simulink model "sim_tcyb_2024_pos_ctrl"  (R2020a)
settings: Solver=ode4  StartTime=0.0  StopTime=30.0  FixedStep=0.01  RelTol=1e-3
values from neighbouring files (symbols this model uses):
  alfa_theta = 20    [init_tcyb_2024_pos_ctrl.m]
  alfa_theta_obs = 100    [init_tcyb_2024_pos_ctrl.m]
  c1_diff_sigma_bar_v = diag([25; 30; 20])    [init_tcyb_2024_pos_ctrl.m]
  c1v = diag([5.8; 6.5; 6.5])    [init_tcyb_2024_pos_ctrl.m]
  c2_diff_sigma_bar_v = diag([50; 50; 10])    [init_tcyb_2024_pos_ctrl.m]
  c2v = diag([5.8; 6.5; 6.5])    [init_tcyb_2024_pos_ctrl.m]
  c3_diff_sigma_bar_v = diag([15; 15; 10])    [init_tcyb_2024_pos_ctrl.m]
  c3v = diag([4.8; 6.4; 6.0])    [init_tcyb_2024_pos_ctrl.m]
  c_psi_p = [0.05; 0.05; 0.05]    [init_tcyb_2024_pos_ctrl.m]
  delta_p_i_0 = zeros(3, NF)    [init_tcyb_2024_pos_ctrl.m]
  delta_v_i_0 = zeros(3, NF)    [init_tcyb_2024_pos_ctrl.m]
  dp_aa_t = 0.2 * ones(3, 5) + ( 1.0 - 0.2 ) * rand(3, 5)    [init_tcyb_2024_pos_ctrl.m]
  dp_ff_t = [ 0.4 * ones(1, 5) + ( 1.0 - 0.4 ) * rand(1, 5);                      0.4 * ones(1, 5) + ( 1.0 - 0.4 ) * rand(1, 5);                      0.2 * ones(1, 5) + ( 0.6 - 0.2 ) * rand(1, 5) ]    [init_tcyb_2024_pos_ctrl.m]
  dp_phi_t = ( - pi / 2 ) * ones(3, 5) + ( pi / 2 - ( - pi / 2 ) ) * rand(3, 5)    [init_tcyb_2024_pos_ctrl.m]
  etai_0 = zeros(3,5)    [init_tcyb_2024_pos_ctrl.m]
  kai_1_t = 0.02    [init_tcyb_2024_pos_ctrl.m]
  kai_3_t = 0.1    [init_tcyb_2024_pos_ctrl.m]
  ksii_0 = zeros(3,5)    [init_tcyb_2024_pos_ctrl.m]
  l1v = diag([20; 20; 20])    [init_tcyb_2024_pos_ctrl.m]
  l2v = diag([30; 30; 30])    [init_tcyb_2024_pos_ctrl.m]
  Lamd_diff_sigma_bar_v = 0.5    [init_tcyb_2024_pos_ctrl.m]
  mass_i = zeros(1,NF)    [init_tcyb_2024_pos_ctrl.m]
  Mii = diag([1;0;0;0;1])    [init_tcyb_2024_pos_ctrl.m]
  pos0 = zeros(3, 1)    [init_tcyb_2024_pos_ctrl.m]
  PZ0 = P0(3)    [init_tcyb_2024_pos_ctrl.m]
  PZ1 = 10    [init_tcyb_2024_pos_ctrl.m]
  Qci_init = repmat([1;0;0;0],1,NF)    [init_tcyb_2024_pos_ctrl.m]
  R0 = 4    [init_tcyb_2024_pos_ctrl.m]
  R1 = 8    [init_tcyb_2024_pos_ctrl.m]
  rho_p = [0.1; 0.1; 0.1]    [init_tcyb_2024_pos_ctrl.m]
  Rx2 = 10    [init_tcyb_2024_pos_ctrl.m]
  Ry2 = 6    [init_tcyb_2024_pos_ctrl.m]
  Rz2 = 4    [init_tcyb_2024_pos_ctrl.m]
  T0 = 0    [init_tcyb_2024_pos_ctrl.m]
  T1 = tseq1    (= 10)    [init_tcyb_2024_pos_ctrl.m]
  T12 = tseq1 + tseq12    (= 20)    [init_tcyb_2024_pos_ctrl.m]
  T2 = tseq1 + tseq12 + tseq2    (= 30)    [init_tcyb_2024_pos_ctrl.m]
  tau_p = 5    [init_tcyb_2024_pos_ctrl.m]
  theta0 = ( 2 / 5 ) * pi    (= 1.25663706144)    [init_tcyb_2024_pos_ctrl.m]
  vel0 = zeros(3, 1)    [init_tcyb_2024_pos_ctrl.m]
  Wij = [0,0,1,0,0;              0,0,1,1,0;              1,0,0,0,1;              0,1,1,0,0;              0,0,1,0,0]    [init_tcyb_2024_pos_ctrl.m]
  X1 = 8    [init_tcyb_2024_pos_ctrl.m]
  X2 = 2    [init_tcyb_2024_pos_ctrl.m]
  X3 = 3    [init_tcyb_2024_pos_ctrl.m]
  Y1 = 10    [init_tcyb_2024_pos_ctrl.m]
  Y2 = 2    [init_tcyb_2024_pos_ctrl.m]
  Y3 = 4    [init_tcyb_2024_pos_ctrl.m]
  Z1 = 4    [init_tcyb_2024_pos_ctrl.m]
  Z2 = -6    [init_tcyb_2024_pos_ctrl.m]
  Z3 = 2    [init_tcyb_2024_pos_ctrl.m]
  zeta_diff_sigma_bar_v = 0.08    [init_tcyb_2024_pos_ctrl.m]
undefined symbols (not defined in the file or in its folder): cal_frac_squ, p_alfav1, p_alfav2, p_gamma1_pos, p_gamma1_vel, p_gamma2_pos, p_gamma2_vel, q_alfav1, q_alfav2, q_gamma1_pos, q_gamma1_vel, q_gamma2_pos, q_gamma2_vel
(part 2 of 4)

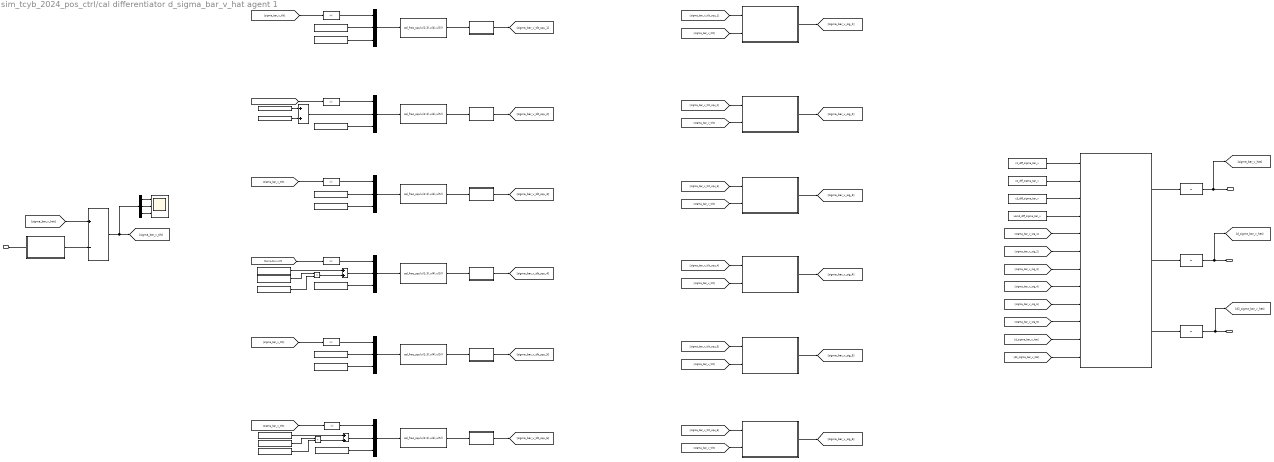
== system sim_tcyb_2024_pos_ctrl/cal differentiator d_sigma_bar_v_hat agent 1 ==
  x : Inport
  Abs{,1..5} (6 alike) : Abs
  Add : Sum
  Add1 : Sum
  Add2 : Sum
  Add3 : Sum  Inputs=+-
  Constant : Constant  Value=0
  Constant{97,100,105,107,109} (5 alike) : Constant
  Constant{98..99,101,108,110..111} (6 alike) : Constant  Value=3
  Constant102 : Constant  Value=2
  Constant103 : Constant  Value=c1_diff_sigma_bar_v
  Constant104 : Constant  Value=c2_diff_sigma_bar_v
  Constant106 : Constant  Value=c3_diff_sigma_bar_v
  Constant112 : Constant  Value=2
  Constant113 : Constant  Value=Lamd_diff_sigma_bar_v
  Constant161 : Constant  Value=zeta_diff_sigma_bar_v
  Constant162 : Constant  Value=zeta_diff_sigma_bar_v
  Constant163 : Constant  Value=zeta_diff_sigma_bar_v
  Demux2 : Demux  Outputs=3
  Integrator2 : Integrator  InitialCondition=zeros(3,1)
  Integrator3 : Integrator  InitialCondition=zeros(3,1)
  Integrator4 : Integrator  InitialCondition=zeros(3,1)
  Interpreted MATLAB Function{,20..24} (6 alike) : MATLABFcn  MATLABFcn=cal_frac_squ(u(1:3),u(4),u(5))
  Mux{19..24} (6 alike) : Mux  Inputs=3
  Product : Product
  Product1 : Product
  cal differentiator : MATLAB Function  TreatAsAtomicUnit=on
  cal sig : MATLAB Function  TreatAsAtomicUnit=on
  cal sig1 : MATLAB Function  TreatAsAtomicUnit=on
  cal sig2 : MATLAB Function  TreatAsAtomicUnit=on
  cal sig3 : MATLAB Function  TreatAsAtomicUnit=on
  cal sig4 : MATLAB Function  TreatAsAtomicUnit=on
  cal sig5 : MATLAB Function  TreatAsAtomicUnit=on
  choose sigma_bar_v : MATLAB Function  TreatAsAtomicUnit=on
  sigma_bar_v_tilt : Scope  NumInputPorts=3
  trans to column20 : MATLAB Function  TreatAsAtomicUnit=on
  trans to column21 : MATLAB Function  TreatAsAtomicUnit=on
  trans to column22 : MATLAB Function  TreatAsAtomicUnit=on
  trans to column23 : MATLAB Function  TreatAsAtomicUnit=on
  trans to column24 : MATLAB Function  TreatAsAtomicUnit=on
  trans to column25 : MATLAB Function  TreatAsAtomicUnit=on
  Out1 : Outport
  Out2 : Outport  Port=2
  Out3 : Outport  Port=3
  wires:
  Abs/1 -> Mux22/1
  [sigma_bar_v_tilt] -> cal sig/2(y)
  cal sig1/1(z) -> [sigma_bar_v_sig_2]
  [d2_sigma_bar_v_hat] -> cal differentiator/12(d2_sigma_bar_v_hat)
  trans to column23/1(y) -> [sigma_bar_v_tilt_squ_3]
  Add/1 -> Mux21/2
  Demux2/1 -> sigma_bar_v_tilt/1
  [sigma_bar_v_tilt] -> cal sig4/2(y)
  Product1/1 -> Add2/2
  Add2/1 -> Mux19/2
  [d_sigma_bar_v_hat] -> cal differentiator/11("d_sigma_bar_v_hat ")
  [sigma_bar_v_sig_3] -> cal differentiator/7(sigma_bar_v_sig_3)
  trans to column24/1(y) -> [sigma_bar_v_tilt_squ_4]
  Constant107/1 -> Mux21/3
  [sigma_bar_v_sig_5] -> cal differentiator/9(sigma_bar_v_sig_5)
  Constant97/1 -> Mux22/3
  cal sig/1(z) -> [sigma_bar_v_sig_1]
  trans to column22/1(y) -> [sigma_bar_v_tilt_squ_1]
  [sigma_bar_v_tilt_squ_3] -> cal sig2/1(x)
  [sigma_bar_v_tilt] -> Abs3/1
  Interpreted MATLAB Function24/1 -> trans to column25/1(x)
  [sigma_bar_v_sig_1] -> cal differentiator/5(sigma_bar_v_sig_1)
  cal differentiator/1(d_sigma_bar_v_hat) -> Integrator2/1
  Constant110/1 -> Mux24/3
  cal sig5/1(z) -> [sigma_bar_v_sig_5]
  [sigma_bar_v_tilt] -> Abs4/1
  Demux2/3 -> sigma_bar_v_tilt/3
  cal sig2/1(z) -> [sigma_bar_v_sig_3]
  Constant112/1 -> Product/1
  Constant/1 -> Mux22/2
  cal differentiator/3(d_d2sigma_bar_v_hat) -> Integrator4/1
  Abs3/1 -> Mux24/1
  trans to column21/1(y) -> [sigma_bar_v_tilt_squ_2]
  Constant99/1 -> Add2/1
  Constant103/1 -> cal differentiator/1(c1)
  Mux19/1 -> Interpreted MATLAB Function24/1
  [sigma_bar_v_tilt_squ_6] -> cal sig3/1(x)
  Constant106/1 -> cal differentiator/3(c3)
  [sigma_bar_v_tilt] -> Abs2/1
  [sigma_bar_v_tilt_squ_2] -> cal sig1/1(x)
  Constant162/1 -> Product/2
  Product/1 -> Add1/2
  [sigma_bar_v_sig_4] -> cal differentiator/8(sigma_bar_v_sig_4)
  [sigma_bar_v_hat] -> Add3/1
  Constant102/1 -> Mux20/2
  Add3/1 -> Demux2/1, [sigma_bar_v_tilt]
  cal differentiator/2(d_dsigma_bar_v_hat) -> Integrator3/1
  [sigma_bar_v_tilt] -> Abs5/1
  [sigma_bar_v_tilt] -> cal sig2/2(y)
  [sigma_bar_v_sig_6] -> cal differentiator/10(sigma_bar_v_sig_6)
  trans to column20/1(y) -> [sigma_bar_v_tilt_squ_5]
  Constant104/1 -> cal differentiator/2(c2)
  Constant101/1 -> Mux20/3
  Mux22/1 -> Interpreted MATLAB Function/1
  Constant163/1 -> Product1/2
  Abs2/1 -> Mux23/1
  Interpreted MATLAB Function21/1 -> trans to column21/1(x)
  Interpreted MATLAB Function23/1 -> trans to column24/1(x)
  Mux23/1 -> Interpreted MATLAB Function22/1
  cal sig3/1(z) -> [sigma_bar_v_sig_6]
  Abs4/1 -> Mux19/1
  trans to column25/1(y) -> [sigma_bar_v_tilt_squ_6]
  Constant113/1 -> cal differentiator/4(chi_t)
  choose sigma_bar_v/1(y) -> Add3/2
  Interpreted MATLAB Function/1 -> trans to column22/1(x)
  Interpreted MATLAB Function20/1 -> trans to column20/1(x)
  Constant108/1 -> Mux23/3
  [sigma_bar_v_sig_2] -> cal differentiator/6(sigma_bar_v_sig_2)
  [sigma_bar_v_tilt] -> cal sig1/2(y)
  [sigma_bar_v_tilt_squ_1] -> cal sig/1(x)
  Constant100/1 -> Product1/1
  Abs1/1 -> Mux21/1
  Demux2/2 -> sigma_bar_v_tilt/2
  Integrator4/1 -> [d2_sigma_bar_v_hat], Out3/1
  [sigma_bar_v_tilt_squ_4] -> cal sig4/1(x)
  Abs5/1 -> Mux20/1
  Constant98/1 -> Mux19/3
  Constant111/1 -> Add1/1
  [sigma_bar_v_tilt] -> cal sig5/2(y)
  Constant109/1 -> Mux23/2
  [sigma_bar_v_tilt] -> Abs/1
  Mux24/1 -> Interpreted MATLAB Function23/1
  [sigma_bar_v_tilt] -> Abs1/1
  [sigma_bar_v_tilt_squ_5] -> cal sig5/1(x)
  Add1/1 -> Mux24/2
  cal sig4/1(z) -> [sigma_bar_v_sig_4]
  Constant161/1 -> Add/2
  [sigma_bar_v_tilt] -> cal sig3/2(y)
  Mux21/1 -> Interpreted MATLAB Function21/1
  Interpreted MATLAB Function22/1 -> trans to column23/1(x)
  Mux20/1 -> Interpreted MATLAB Function20/1
  x/1 -> choose sigma_bar_v/1(x)
  Constant105/1 -> Add/1
  Integrator2/1 -> [sigma_bar_v_hat], Out1/1
  Integrator3/1 -> [d_sigma_bar_v_hat], Out2/1

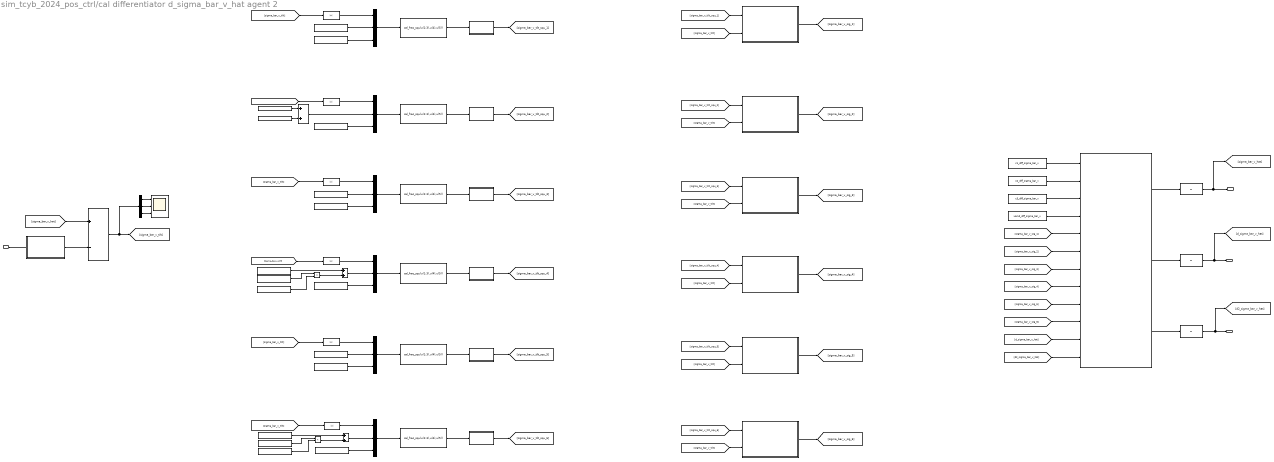
== system sim_tcyb_2024_pos_ctrl/cal differentiator d_sigma_bar_v_hat agent 2 ==
  x : Inport
  Abs{,1..5} (6 alike) : Abs
  Add : Sum
  Add1 : Sum
  Add2 : Sum
  Add3 : Sum  Inputs=+-
  Constant : Constant  Value=0
  Constant{97,100,105,107,109} (5 alike) : Constant
  Constant{98..99,101,108,110..111} (6 alike) : Constant  Value=3
  Constant102 : Constant  Value=2
  Constant103 : Constant  Value=c1_diff_sigma_bar_v
  Constant104 : Constant  Value=c2_diff_sigma_bar_v
  Constant106 : Constant  Value=c3_diff_sigma_bar_v
  Constant112 : Constant  Value=2
  Constant113 : Constant  Value=Lamd_diff_sigma_bar_v
  Constant161 : Constant  Value=zeta_diff_sigma_bar_v
  Constant162 : Constant  Value=zeta_diff_sigma_bar_v
  Constant163 : Constant  Value=zeta_diff_sigma_bar_v
  Demux2 : Demux  Outputs=3
  Integrator2 : Integrator  InitialCondition=zeros(3,1)
  Integrator3 : Integrator  InitialCondition=zeros(3,1)
  Integrator4 : Integrator  InitialCondition=zeros(3,1)
  Interpreted MATLAB Function{,20..24} (6 alike) : MATLABFcn  MATLABFcn=cal_frac_squ(u(1:3),u(4),u(5))
  Mux{19..24} (6 alike) : Mux  Inputs=3
  Product : Product
  Product1 : Product
  cal differentiator : MATLAB Function  TreatAsAtomicUnit=on
  cal sig : MATLAB Function  TreatAsAtomicUnit=on
  cal sig1 : MATLAB Function  TreatAsAtomicUnit=on
  cal sig2 : MATLAB Function  TreatAsAtomicUnit=on
  cal sig3 : MATLAB Function  TreatAsAtomicUnit=on
  cal sig4 : MATLAB Function  TreatAsAtomicUnit=on
  cal sig5 : MATLAB Function  TreatAsAtomicUnit=on
  choose sigma_bar_v : MATLAB Function  TreatAsAtomicUnit=on
  sigma_bar_v_tilt : Scope  NumInputPorts=3
  trans to column20 : MATLAB Function  TreatAsAtomicUnit=on
  trans to column21 : MATLAB Function  TreatAsAtomicUnit=on
  trans to column22 : MATLAB Function  TreatAsAtomicUnit=on
  trans to column23 : MATLAB Function  TreatAsAtomicUnit=on
  trans to column24 : MATLAB Function  TreatAsAtomicUnit=on
  trans to column25 : MATLAB Function  TreatAsAtomicUnit=on
  Out1 : Outport
  Out2 : Outport  Port=2
  Out3 : Outport  Port=3
  wires:
  Abs/1 -> Mux22/1
  [sigma_bar_v_tilt] -> cal sig/2(y)
  cal sig1/1(z) -> [sigma_bar_v_sig_2]
  [d2_sigma_bar_v_hat] -> cal differentiator/12(d2_sigma_bar_v_hat)
  trans to column23/1(y) -> [sigma_bar_v_tilt_squ_3]
  Add/1 -> Mux21/2
  Demux2/1 -> sigma_bar_v_tilt/1
  [sigma_bar_v_tilt] -> cal sig4/2(y)
  Product1/1 -> Add2/2
  Add2/1 -> Mux19/2
  [d_sigma_bar_v_hat] -> cal differentiator/11("d_sigma_bar_v_hat ")
  [sigma_bar_v_sig_3] -> cal differentiator/7(sigma_bar_v_sig_3)
  trans to column24/1(y) -> [sigma_bar_v_tilt_squ_4]
  Constant107/1 -> Mux21/3
  [sigma_bar_v_sig_5] -> cal differentiator/9(sigma_bar_v_sig_5)
  Constant97/1 -> Mux22/3
  cal sig/1(z) -> [sigma_bar_v_sig_1]
  trans to column22/1(y) -> [sigma_bar_v_tilt_squ_1]
  [sigma_bar_v_tilt_squ_3] -> cal sig2/1(x)
  [sigma_bar_v_tilt] -> Abs3/1
  Interpreted MATLAB Function24/1 -> trans to column25/1(x)
  [sigma_bar_v_sig_1] -> cal differentiator/5(sigma_bar_v_sig_1)
  cal differentiator/1(d_sigma_bar_v_hat) -> Integrator2/1
  Constant110/1 -> Mux24/3
  cal sig5/1(z) -> [sigma_bar_v_sig_5]
  [sigma_bar_v_tilt] -> Abs4/1
  Demux2/3 -> sigma_bar_v_tilt/3
  cal sig2/1(z) -> [sigma_bar_v_sig_3]
  Constant112/1 -> Product/1
  Constant/1 -> Mux22/2
  cal differentiator/3(d_d2sigma_bar_v_hat) -> Integrator4/1
  Abs3/1 -> Mux24/1
  trans to column21/1(y) -> [sigma_bar_v_tilt_squ_2]
  Constant99/1 -> Add2/1
  Constant103/1 -> cal differentiator/1(c1)
  Mux19/1 -> Interpreted MATLAB Function24/1
  [sigma_bar_v_tilt_squ_6] -> cal sig3/1(x)
  Constant106/1 -> cal differentiator/3(c3)
  [sigma_bar_v_tilt] -> Abs2/1
  [sigma_bar_v_tilt_squ_2] -> cal sig1/1(x)
  Constant162/1 -> Product/2
  Product/1 -> Add1/2
  [sigma_bar_v_sig_4] -> cal differentiator/8(sigma_bar_v_sig_4)
  [sigma_bar_v_hat] -> Add3/1
  Constant102/1 -> Mux20/2
  Add3/1 -> Demux2/1, [sigma_bar_v_tilt]
  cal differentiator/2(d_dsigma_bar_v_hat) -> Integrator3/1
  [sigma_bar_v_tilt] -> Abs5/1
  [sigma_bar_v_tilt] -> cal sig2/2(y)
  [sigma_bar_v_sig_6] -> cal differentiator/10(sigma_bar_v_sig_6)
  trans to column20/1(y) -> [sigma_bar_v_tilt_squ_5]
  Constant104/1 -> cal differentiator/2(c2)
  Constant101/1 -> Mux20/3
  Mux22/1 -> Interpreted MATLAB Function/1
  Constant163/1 -> Product1/2
  Abs2/1 -> Mux23/1
  Interpreted MATLAB Function21/1 -> trans to column21/1(x)
  Interpreted MATLAB Function23/1 -> trans to column24/1(x)
  Mux23/1 -> Interpreted MATLAB Function22/1
  cal sig3/1(z) -> [sigma_bar_v_sig_6]
  Abs4/1 -> Mux19/1
  trans to column25/1(y) -> [sigma_bar_v_tilt_squ_6]
  Constant113/1 -> cal differentiator/4(chi_t)
  choose sigma_bar_v/1(y) -> Add3/2
  Interpreted MATLAB Function/1 -> trans to column22/1(x)
  Interpreted MATLAB Function20/1 -> trans to column20/1(x)
  Constant108/1 -> Mux23/3
  [sigma_bar_v_sig_2] -> cal differentiator/6(sigma_bar_v_sig_2)
  [sigma_bar_v_tilt] -> cal sig1/2(y)
  [sigma_bar_v_tilt_squ_1] -> cal sig/1(x)
  Constant100/1 -> Product1/1
  Abs1/1 -> Mux21/1
  Demux2/2 -> sigma_bar_v_tilt/2
  Integrator4/1 -> [d2_sigma_bar_v_hat], Out3/1
  [sigma_bar_v_tilt_squ_4] -> cal sig4/1(x)
  Abs5/1 -> Mux20/1
  Constant98/1 -> Mux19/3
  Constant111/1 -> Add1/1
  [sigma_bar_v_tilt] -> cal sig5/2(y)
  Constant109/1 -> Mux23/2
  [sigma_bar_v_tilt] -> Abs/1
  Mux24/1 -> Interpreted MATLAB Function23/1
  [sigma_bar_v_tilt] -> Abs1/1
  [sigma_bar_v_tilt_squ_5] -> cal sig5/1(x)
  Add1/1 -> Mux24/2
  cal sig4/1(z) -> [sigma_bar_v_sig_4]
  Constant161/1 -> Add/2
  [sigma_bar_v_tilt] -> cal sig3/2(y)
  Mux21/1 -> Interpreted MATLAB Function21/1
  Interpreted MATLAB Function22/1 -> trans to column23/1(x)
  Mux20/1 -> Interpreted MATLAB Function20/1
  x/1 -> choose sigma_bar_v/1(x)
  Constant105/1 -> Add/1
  Integrator2/1 -> [sigma_bar_v_hat], Out1/1
  Integrator3/1 -> [d_sigma_bar_v_hat], Out2/1

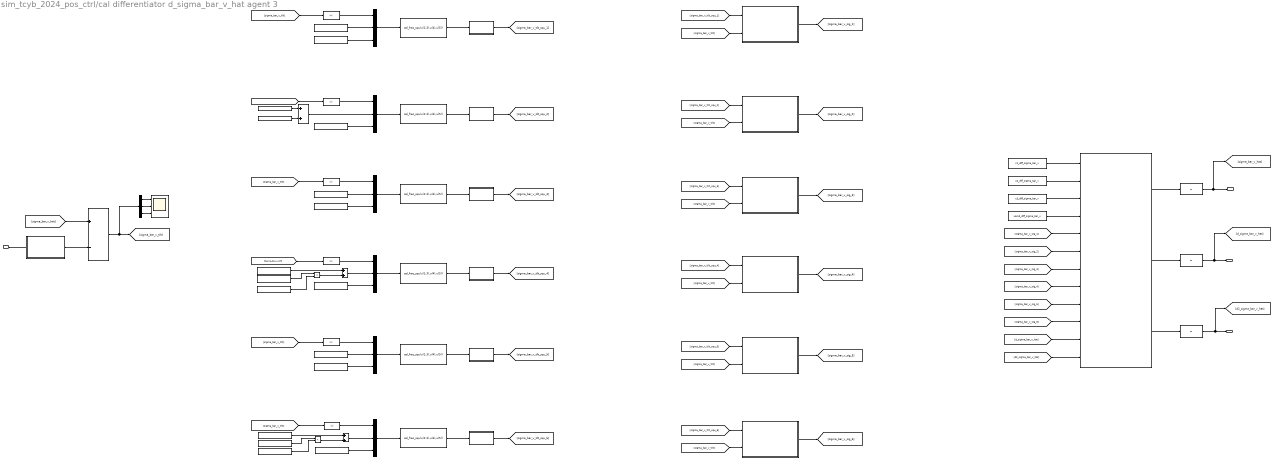
== system sim_tcyb_2024_pos_ctrl/cal differentiator d_sigma_bar_v_hat agent 3 ==
  x : Inport
  Abs{,1..5} (6 alike) : Abs
  Add : Sum
  Add1 : Sum
  Add2 : Sum
  Add3 : Sum  Inputs=+-
  Constant : Constant  Value=0
  Constant{97,100,105,107,109} (5 alike) : Constant
  Constant{98..99,101,108,110..111} (6 alike) : Constant  Value=3
  Constant102 : Constant  Value=2
  Constant103 : Constant  Value=c1_diff_sigma_bar_v
  Constant104 : Constant  Value=c2_diff_sigma_bar_v
  Constant106 : Constant  Value=c3_diff_sigma_bar_v
  Constant112 : Constant  Value=2
  Constant113 : Constant  Value=Lamd_diff_sigma_bar_v
  Constant161 : Constant  Value=zeta_diff_sigma_bar_v
  Constant162 : Constant  Value=zeta_diff_sigma_bar_v
  Constant163 : Constant  Value=zeta_diff_sigma_bar_v
  Demux2 : Demux  Outputs=3
  Integrator2 : Integrator  InitialCondition=zeros(3,1)
  Integrator3 : Integrator  InitialCondition=zeros(3,1)
  Integrator4 : Integrator  InitialCondition=zeros(3,1)
  Interpreted MATLAB Function{,20..24} (6 alike) : MATLABFcn  MATLABFcn=cal_frac_squ(u(1:3),u(4),u(5))
  Mux{19..24} (6 alike) : Mux  Inputs=3
  Product : Product
  Product1 : Product
  cal differentiator : MATLAB Function  TreatAsAtomicUnit=on
  cal sig : MATLAB Function  TreatAsAtomicUnit=on
  cal sig1 : MATLAB Function  TreatAsAtomicUnit=on
  cal sig2 : MATLAB Function  TreatAsAtomicUnit=on
  cal sig3 : MATLAB Function  TreatAsAtomicUnit=on
  cal sig4 : MATLAB Function  TreatAsAtomicUnit=on
  cal sig5 : MATLAB Function  TreatAsAtomicUnit=on
  choose sigma_bar_v : MATLAB Function  TreatAsAtomicUnit=on
  sigma_bar_v_tilt : Scope  NumInputPorts=3
  trans to column20 : MATLAB Function  TreatAsAtomicUnit=on
  trans to column21 : MATLAB Function  TreatAsAtomicUnit=on
  trans to column22 : MATLAB Function  TreatAsAtomicUnit=on
  trans to column23 : MATLAB Function  TreatAsAtomicUnit=on
  trans to column24 : MATLAB Function  TreatAsAtomicUnit=on
  trans to column25 : MATLAB Function  TreatAsAtomicUnit=on
  Out1 : Outport
  Out2 : Outport  Port=2
  Out3 : Outport  Port=3
  wires:
  Abs/1 -> Mux22/1
  [sigma_bar_v_tilt] -> cal sig/2(y)
  cal sig1/1(z) -> [sigma_bar_v_sig_2]
  [d2_sigma_bar_v_hat] -> cal differentiator/12(d2_sigma_bar_v_hat)
  trans to column23/1(y) -> [sigma_bar_v_tilt_squ_3]
  Add/1 -> Mux21/2
  Demux2/1 -> sigma_bar_v_tilt/1
  [sigma_bar_v_tilt] -> cal sig4/2(y)
  Product1/1 -> Add2/2
  Add2/1 -> Mux19/2
  [d_sigma_bar_v_hat] -> cal differentiator/11("d_sigma_bar_v_hat ")
  [sigma_bar_v_sig_3] -> cal differentiator/7(sigma_bar_v_sig_3)
  trans to column24/1(y) -> [sigma_bar_v_tilt_squ_4]
  Constant107/1 -> Mux21/3
  [sigma_bar_v_sig_5] -> cal differentiator/9(sigma_bar_v_sig_5)
  Constant97/1 -> Mux22/3
  cal sig/1(z) -> [sigma_bar_v_sig_1]
  trans to column22/1(y) -> [sigma_bar_v_tilt_squ_1]
  [sigma_bar_v_tilt_squ_3] -> cal sig2/1(x)
  [sigma_bar_v_tilt] -> Abs3/1
  Interpreted MATLAB Function24/1 -> trans to column25/1(x)
  [sigma_bar_v_sig_1] -> cal differentiator/5(sigma_bar_v_sig_1)
  cal differentiator/1(d_sigma_bar_v_hat) -> Integrator2/1
  Constant110/1 -> Mux24/3
  cal sig5/1(z) -> [sigma_bar_v_sig_5]
  [sigma_bar_v_tilt] -> Abs4/1
  Demux2/3 -> sigma_bar_v_tilt/3
  cal sig2/1(z) -> [sigma_bar_v_sig_3]
  Constant112/1 -> Product/1
  Constant/1 -> Mux22/2
  cal differentiator/3(d_d2sigma_bar_v_hat) -> Integrator4/1
  Abs3/1 -> Mux24/1
  trans to column21/1(y) -> [sigma_bar_v_tilt_squ_2]
  Constant99/1 -> Add2/1
  Constant103/1 -> cal differentiator/1(c1)
  Mux19/1 -> Interpreted MATLAB Function24/1
  [sigma_bar_v_tilt_squ_6] -> cal sig3/1(x)
  Constant106/1 -> cal differentiator/3(c3)
  [sigma_bar_v_tilt] -> Abs2/1
  [sigma_bar_v_tilt_squ_2] -> cal sig1/1(x)
  Constant162/1 -> Product/2
  Product/1 -> Add1/2
  [sigma_bar_v_sig_4] -> cal differentiator/8(sigma_bar_v_sig_4)
  [sigma_bar_v_hat] -> Add3/1
  Constant102/1 -> Mux20/2
  Add3/1 -> Demux2/1, [sigma_bar_v_tilt]
  cal differentiator/2(d_dsigma_bar_v_hat) -> Integrator3/1
  [sigma_bar_v_tilt] -> Abs5/1
  [sigma_bar_v_tilt] -> cal sig2/2(y)
  [sigma_bar_v_sig_6] -> cal differentiator/10(sigma_bar_v_sig_6)
  trans to column20/1(y) -> [sigma_bar_v_tilt_squ_5]
  Constant104/1 -> cal differentiator/2(c2)
  Constant101/1 -> Mux20/3
  Mux22/1 -> Interpreted MATLAB Function/1
  Constant163/1 -> Product1/2
  Abs2/1 -> Mux23/1
  Interpreted MATLAB Function21/1 -> trans to column21/1(x)
  Interpreted MATLAB Function23/1 -> trans to column24/1(x)
  Mux23/1 -> Interpreted MATLAB Function22/1
  cal sig3/1(z) -> [sigma_bar_v_sig_6]
  Abs4/1 -> Mux19/1
  trans to column25/1(y) -> [sigma_bar_v_tilt_squ_6]
  Constant113/1 -> cal differentiator/4(chi_t)
  choose sigma_bar_v/1(y) -> Add3/2
  Interpreted MATLAB Function/1 -> trans to column22/1(x)
  Interpreted MATLAB Function20/1 -> trans to column20/1(x)
  Constant108/1 -> Mux23/3
  [sigma_bar_v_sig_2] -> cal differentiator/6(sigma_bar_v_sig_2)
  [sigma_bar_v_tilt] -> cal sig1/2(y)
  [sigma_bar_v_tilt_squ_1] -> cal sig/1(x)
  Constant100/1 -> Product1/1
  Abs1/1 -> Mux21/1
  Demux2/2 -> sigma_bar_v_tilt/2
  Integrator4/1 -> [d2_sigma_bar_v_hat], Out3/1
  [sigma_bar_v_tilt_squ_4] -> cal sig4/1(x)
  Abs5/1 -> Mux20/1
  Constant98/1 -> Mux19/3
  Constant111/1 -> Add1/1
  [sigma_bar_v_tilt] -> cal sig5/2(y)
  Constant109/1 -> Mux23/2
  [sigma_bar_v_tilt] -> Abs/1
  Mux24/1 -> Interpreted MATLAB Function23/1
  [sigma_bar_v_tilt] -> Abs1/1
  [sigma_bar_v_tilt_squ_5] -> cal sig5/1(x)
  Add1/1 -> Mux24/2
  cal sig4/1(z) -> [sigma_bar_v_sig_4]
  Constant161/1 -> Add/2
  [sigma_bar_v_tilt] -> cal sig3/2(y)
  Mux21/1 -> Interpreted MATLAB Function21/1
  Interpreted MATLAB Function22/1 -> trans to column23/1(x)
  Mux20/1 -> Interpreted MATLAB Function20/1
  x/1 -> choose sigma_bar_v/1(x)
  Constant105/1 -> Add/1
  Integrator2/1 -> [sigma_bar_v_hat], Out1/1
  Integrator3/1 -> [d_sigma_bar_v_hat], Out2/1

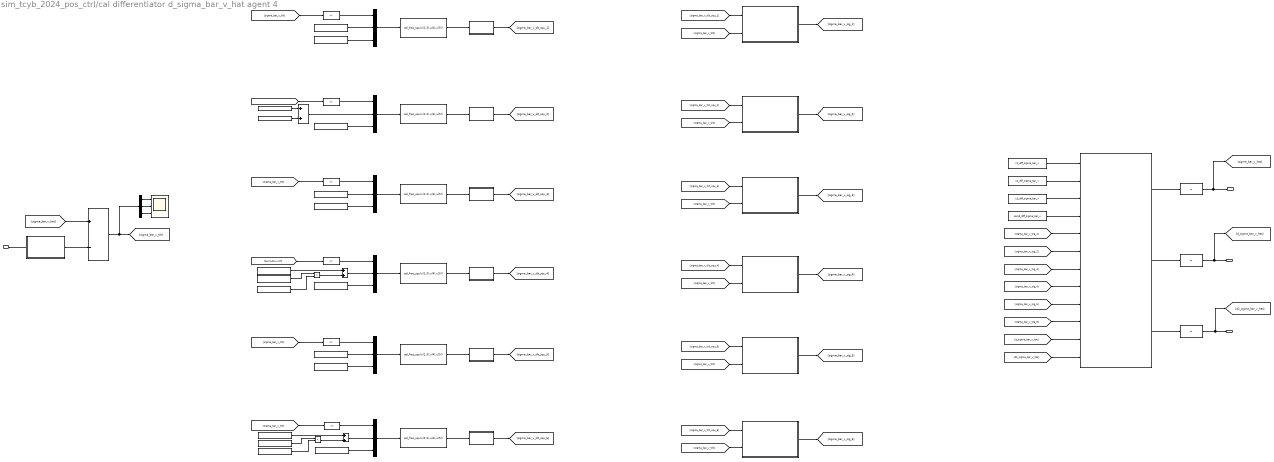
== system sim_tcyb_2024_pos_ctrl/cal differentiator d_sigma_bar_v_hat agent 4 ==
  x : Inport
  Abs{,1..5} (6 alike) : Abs
  Add : Sum
  Add1 : Sum
  Add2 : Sum
  Add3 : Sum  Inputs=+-
  Constant : Constant  Value=0
  Constant{97,100,105,107,109} (5 alike) : Constant
  Constant{98..99,101,108,110..111} (6 alike) : Constant  Value=3
  Constant102 : Constant  Value=2
  Constant103 : Constant  Value=c1_diff_sigma_bar_v
  Constant104 : Constant  Value=c2_diff_sigma_bar_v
  Constant106 : Constant  Value=c3_diff_sigma_bar_v
  Constant112 : Constant  Value=2
  Constant113 : Constant  Value=Lamd_diff_sigma_bar_v
  Constant161 : Constant  Value=zeta_diff_sigma_bar_v
  Constant162 : Constant  Value=zeta_diff_sigma_bar_v
  Constant163 : Constant  Value=zeta_diff_sigma_bar_v
  Demux2 : Demux  Outputs=3
  Integrator2 : Integrator  InitialCondition=zeros(3,1)
  Integrator3 : Integrator  InitialCondition=zeros(3,1)
  Integrator4 : Integrator  InitialCondition=zeros(3,1)
  Interpreted MATLAB Function{,20..24} (6 alike) : MATLABFcn  MATLABFcn=cal_frac_squ(u(1:3),u(4),u(5))
  Mux{19..24} (6 alike) : Mux  Inputs=3
  Product : Product
  Product1 : Product
  cal differentiator : MATLAB Function  TreatAsAtomicUnit=on
  cal sig : MATLAB Function  TreatAsAtomicUnit=on
  cal sig1 : MATLAB Function  TreatAsAtomicUnit=on
  cal sig2 : MATLAB Function  TreatAsAtomicUnit=on
  cal sig3 : MATLAB Function  TreatAsAtomicUnit=on
  cal sig4 : MATLAB Function  TreatAsAtomicUnit=on
  cal sig5 : MATLAB Function  TreatAsAtomicUnit=on
  choose sigma_bar_v : MATLAB Function  TreatAsAtomicUnit=on
  sigma_bar_v_tilt : Scope  NumInputPorts=3
  trans to column20 : MATLAB Function  TreatAsAtomicUnit=on
  trans to column21 : MATLAB Function  TreatAsAtomicUnit=on
  trans to column22 : MATLAB Function  TreatAsAtomicUnit=on
  trans to column23 : MATLAB Function  TreatAsAtomicUnit=on
  trans to column24 : MATLAB Function  TreatAsAtomicUnit=on
  trans to column25 : MATLAB Function  TreatAsAtomicUnit=on
  Out1 : Outport
  Out2 : Outport  Port=2
  Out3 : Outport  Port=3
  wires:
  Abs/1 -> Mux22/1
  [sigma_bar_v_tilt] -> cal sig/2(y)
  cal sig1/1(z) -> [sigma_bar_v_sig_2]
  [d2_sigma_bar_v_hat] -> cal differentiator/12(d2_sigma_bar_v_hat)
  trans to column23/1(y) -> [sigma_bar_v_tilt_squ_3]
  Add/1 -> Mux21/2
  Demux2/1 -> sigma_bar_v_tilt/1
  [sigma_bar_v_tilt] -> cal sig4/2(y)
  Product1/1 -> Add2/2
  Add2/1 -> Mux19/2
  [d_sigma_bar_v_hat] -> cal differentiator/11("d_sigma_bar_v_hat ")
  [sigma_bar_v_sig_3] -> cal differentiator/7(sigma_bar_v_sig_3)
  trans to column24/1(y) -> [sigma_bar_v_tilt_squ_4]
  Constant107/1 -> Mux21/3
  [sigma_bar_v_sig_5] -> cal differentiator/9(sigma_bar_v_sig_5)
  Constant97/1 -> Mux22/3
  cal sig/1(z) -> [sigma_bar_v_sig_1]
  trans to column22/1(y) -> [sigma_bar_v_tilt_squ_1]
  [sigma_bar_v_tilt_squ_3] -> cal sig2/1(x)
  [sigma_bar_v_tilt] -> Abs3/1
  Interpreted MATLAB Function24/1 -> trans to column25/1(x)
  [sigma_bar_v_sig_1] -> cal differentiator/5(sigma_bar_v_sig_1)
  cal differentiator/1(d_sigma_bar_v_hat) -> Integrator2/1
  Constant110/1 -> Mux24/3
  cal sig5/1(z) -> [sigma_bar_v_sig_5]
  [sigma_bar_v_tilt] -> Abs4/1
  Demux2/3 -> sigma_bar_v_tilt/3
  cal sig2/1(z) -> [sigma_bar_v_sig_3]
  Constant112/1 -> Product/1
  Constant/1 -> Mux22/2
  cal differentiator/3(d_d2sigma_bar_v_hat) -> Integrator4/1
  Abs3/1 -> Mux24/1
  trans to column21/1(y) -> [sigma_bar_v_tilt_squ_2]
  Constant99/1 -> Add2/1
  Constant103/1 -> cal differentiator/1(c1)
  Mux19/1 -> Interpreted MATLAB Function24/1
  [sigma_bar_v_tilt_squ_6] -> cal sig3/1(x)
  Constant106/1 -> cal differentiator/3(c3)
  [sigma_bar_v_tilt] -> Abs2/1
  [sigma_bar_v_tilt_squ_2] -> cal sig1/1(x)
  Constant162/1 -> Product/2
  Product/1 -> Add1/2
  [sigma_bar_v_sig_4] -> cal differentiator/8(sigma_bar_v_sig_4)
  [sigma_bar_v_hat] -> Add3/1
  Constant102/1 -> Mux20/2
  Add3/1 -> Demux2/1, [sigma_bar_v_tilt]
  cal differentiator/2(d_dsigma_bar_v_hat) -> Integrator3/1
  [sigma_bar_v_tilt] -> Abs5/1
  [sigma_bar_v_tilt] -> cal sig2/2(y)
  [sigma_bar_v_sig_6] -> cal differentiator/10(sigma_bar_v_sig_6)
  trans to column20/1(y) -> [sigma_bar_v_tilt_squ_5]
  Constant104/1 -> cal differentiator/2(c2)
  Constant101/1 -> Mux20/3
  Mux22/1 -> Interpreted MATLAB Function/1
  Constant163/1 -> Product1/2
  Abs2/1 -> Mux23/1
  Interpreted MATLAB Function21/1 -> trans to column21/1(x)
  Interpreted MATLAB Function23/1 -> trans to column24/1(x)
  Mux23/1 -> Interpreted MATLAB Function22/1
  cal sig3/1(z) -> [sigma_bar_v_sig_6]
  Abs4/1 -> Mux19/1
  trans to column25/1(y) -> [sigma_bar_v_tilt_squ_6]
  Constant113/1 -> cal differentiator/4(chi_t)
  choose sigma_bar_v/1(y) -> Add3/2
  Interpreted MATLAB Function/1 -> trans to column22/1(x)
  Interpreted MATLAB Function20/1 -> trans to column20/1(x)
  Constant108/1 -> Mux23/3
  [sigma_bar_v_sig_2] -> cal differentiator/6(sigma_bar_v_sig_2)
  [sigma_bar_v_tilt] -> cal sig1/2(y)
  [sigma_bar_v_tilt_squ_1] -> cal sig/1(x)
  Constant100/1 -> Product1/1
  Abs1/1 -> Mux21/1
  Demux2/2 -> sigma_bar_v_tilt/2
  Integrator4/1 -> [d2_sigma_bar_v_hat], Out3/1
  [sigma_bar_v_tilt_squ_4] -> cal sig4/1(x)
  Abs5/1 -> Mux20/1
  Constant98/1 -> Mux19/3
  Constant111/1 -> Add1/1
  [sigma_bar_v_tilt] -> cal sig5/2(y)
  Constant109/1 -> Mux23/2
  [sigma_bar_v_tilt] -> Abs/1
  Mux24/1 -> Interpreted MATLAB Function23/1
  [sigma_bar_v_tilt] -> Abs1/1
  [sigma_bar_v_tilt_squ_5] -> cal sig5/1(x)
  Add1/1 -> Mux24/2
  cal sig4/1(z) -> [sigma_bar_v_sig_4]
  Constant161/1 -> Add/2
  [sigma_bar_v_tilt] -> cal sig3/2(y)
  Mux21/1 -> Interpreted MATLAB Function21/1
  Interpreted MATLAB Function22/1 -> trans to column23/1(x)
  Mux20/1 -> Interpreted MATLAB Function20/1
  x/1 -> choose sigma_bar_v/1(x)
  Constant105/1 -> Add/1
  Integrator2/1 -> [sigma_bar_v_hat], Out1/1
  Integrator3/1 -> [d_sigma_bar_v_hat], Out2/1

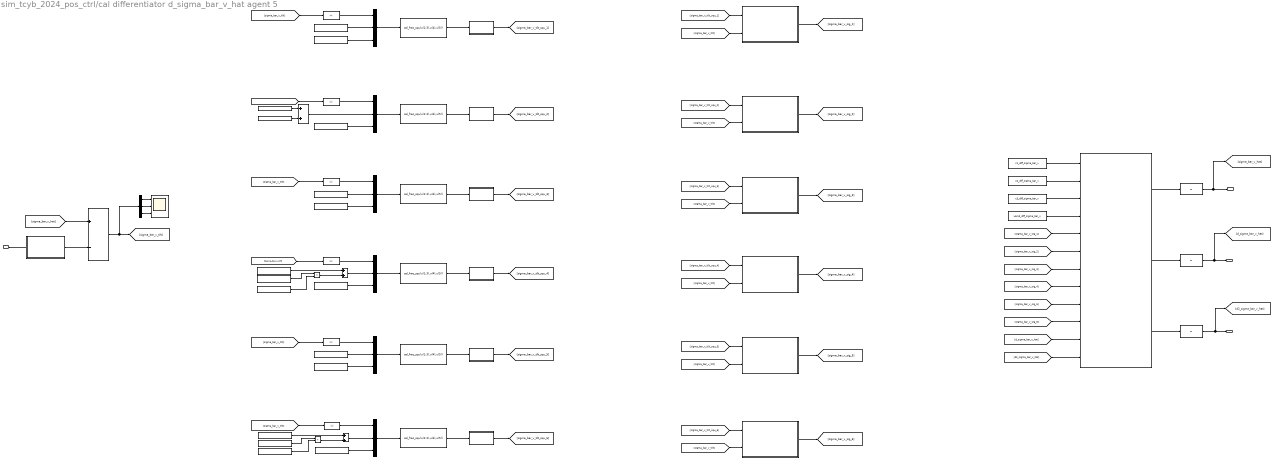
== system sim_tcyb_2024_pos_ctrl/cal differentiator d_sigma_bar_v_hat agent 5 ==
  x : Inport
  Abs{,1..5} (6 alike) : Abs
  Add : Sum
  Add1 : Sum
  Add2 : Sum
  Add3 : Sum  Inputs=+-
  Constant : Constant  Value=0
  Constant{97,100,105,107,109} (5 alike) : Constant
  Constant{98..99,101,108,110..111} (6 alike) : Constant  Value=3
  Constant102 : Constant  Value=2
  Constant103 : Constant  Value=c1_diff_sigma_bar_v
  Constant104 : Constant  Value=c2_diff_sigma_bar_v
  Constant106 : Constant  Value=c3_diff_sigma_bar_v
  Constant112 : Constant  Value=2
  Constant113 : Constant  Value=Lamd_diff_sigma_bar_v
  Constant161 : Constant  Value=zeta_diff_sigma_bar_v
  Constant162 : Constant  Value=zeta_diff_sigma_bar_v
  Constant163 : Constant  Value=zeta_diff_sigma_bar_v
  Demux2 : Demux  Outputs=3
  Integrator2 : Integrator  InitialCondition=zeros(3,1)
  Integrator3 : Integrator  InitialCondition=zeros(3,1)
  Integrator4 : Integrator  InitialCondition=zeros(3,1)
  Interpreted MATLAB Function{,20..24} (6 alike) : MATLABFcn  MATLABFcn=cal_frac_squ(u(1:3),u(4),u(5))
  Mux{19..24} (6 alike) : Mux  Inputs=3
  Product : Product
  Product1 : Product
  cal differentiator : MATLAB Function  TreatAsAtomicUnit=on
  cal sig : MATLAB Function  TreatAsAtomicUnit=on
  cal sig1 : MATLAB Function  TreatAsAtomicUnit=on
  cal sig2 : MATLAB Function  TreatAsAtomicUnit=on
  cal sig3 : MATLAB Function  TreatAsAtomicUnit=on
  cal sig4 : MATLAB Function  TreatAsAtomicUnit=on
  cal sig5 : MATLAB Function  TreatAsAtomicUnit=on
  choose sigma_bar_v : MATLAB Function  TreatAsAtomicUnit=on
  sigma_bar_v_tilt : Scope  NumInputPorts=3
  trans to column20 : MATLAB Function  TreatAsAtomicUnit=on
  trans to column21 : MATLAB Function  TreatAsAtomicUnit=on
  trans to column22 : MATLAB Function  TreatAsAtomicUnit=on
  trans to column23 : MATLAB Function  TreatAsAtomicUnit=on
  trans to column24 : MATLAB Function  TreatAsAtomicUnit=on
  trans to column25 : MATLAB Function  TreatAsAtomicUnit=on
  Out1 : Outport
  Out2 : Outport  Port=2
  Out3 : Outport  Port=3
  wires:
  Abs/1 -> Mux22/1
  [sigma_bar_v_tilt] -> cal sig/2(y)
  cal sig1/1(z) -> [sigma_bar_v_sig_2]
  [d2_sigma_bar_v_hat] -> cal differentiator/12(d2_sigma_bar_v_hat)
  trans to column23/1(y) -> [sigma_bar_v_tilt_squ_3]
  Add/1 -> Mux21/2
  Demux2/1 -> sigma_bar_v_tilt/1
  [sigma_bar_v_tilt] -> cal sig4/2(y)
  Product1/1 -> Add2/2
  Add2/1 -> Mux19/2
  [d_sigma_bar_v_hat] -> cal differentiator/11("d_sigma_bar_v_hat ")
  [sigma_bar_v_sig_3] -> cal differentiator/7(sigma_bar_v_sig_3)
  trans to column24/1(y) -> [sigma_bar_v_tilt_squ_4]
  Constant107/1 -> Mux21/3
  [sigma_bar_v_sig_5] -> cal differentiator/9(sigma_bar_v_sig_5)
  Constant97/1 -> Mux22/3
  cal sig/1(z) -> [sigma_bar_v_sig_1]
  trans to column22/1(y) -> [sigma_bar_v_tilt_squ_1]
  [sigma_bar_v_tilt_squ_3] -> cal sig2/1(x)
  [sigma_bar_v_tilt] -> Abs3/1
  Interpreted MATLAB Function24/1 -> trans to column25/1(x)
  [sigma_bar_v_sig_1] -> cal differentiator/5(sigma_bar_v_sig_1)
  cal differentiator/1(d_sigma_bar_v_hat) -> Integrator2/1
  Constant110/1 -> Mux24/3
  cal sig5/1(z) -> [sigma_bar_v_sig_5]
  [sigma_bar_v_tilt] -> Abs4/1
  Demux2/3 -> sigma_bar_v_tilt/3
  cal sig2/1(z) -> [sigma_bar_v_sig_3]
  Constant112/1 -> Product/1
  Constant/1 -> Mux22/2
  cal differentiator/3(d_d2sigma_bar_v_hat) -> Integrator4/1
  Abs3/1 -> Mux24/1
  trans to column21/1(y) -> [sigma_bar_v_tilt_squ_2]
  Constant99/1 -> Add2/1
  Constant103/1 -> cal differentiator/1(c1)
  Mux19/1 -> Interpreted MATLAB Function24/1
  [sigma_bar_v_tilt_squ_6] -> cal sig3/1(x)
  Constant106/1 -> cal differentiator/3(c3)
  [sigma_bar_v_tilt] -> Abs2/1
  [sigma_bar_v_tilt_squ_2] -> cal sig1/1(x)
  Constant162/1 -> Product/2
  Product/1 -> Add1/2
  [sigma_bar_v_sig_4] -> cal differentiator/8(sigma_bar_v_sig_4)
  [sigma_bar_v_hat] -> Add3/1
  Constant102/1 -> Mux20/2
  Add3/1 -> Demux2/1, [sigma_bar_v_tilt]
  cal differentiator/2(d_dsigma_bar_v_hat) -> Integrator3/1
  [sigma_bar_v_tilt] -> Abs5/1
  [sigma_bar_v_tilt] -> cal sig2/2(y)
  [sigma_bar_v_sig_6] -> cal differentiator/10(sigma_bar_v_sig_6)
  trans to column20/1(y) -> [sigma_bar_v_tilt_squ_5]
  Constant104/1 -> cal differentiator/2(c2)
  Constant101/1 -> Mux20/3
  Mux22/1 -> Interpreted MATLAB Function/1
  Constant163/1 -> Product1/2
  Abs2/1 -> Mux23/1
  Interpreted MATLAB Function21/1 -> trans to column21/1(x)
  Interpreted MATLAB Function23/1 -> trans to column24/1(x)
  Mux23/1 -> Interpreted MATLAB Function22/1
  cal sig3/1(z) -> [sigma_bar_v_sig_6]
  Abs4/1 -> Mux19/1
  trans to column25/1(y) -> [sigma_bar_v_tilt_squ_6]
  Constant113/1 -> cal differentiator/4(chi_t)
  choose sigma_bar_v/1(y) -> Add3/2
  Interpreted MATLAB Function/1 -> trans to column22/1(x)
  Interpreted MATLAB Function20/1 -> trans to column20/1(x)
  Constant108/1 -> Mux23/3
  [sigma_bar_v_sig_2] -> cal differentiator/6(sigma_bar_v_sig_2)
  [sigma_bar_v_tilt] -> cal sig1/2(y)
  [sigma_bar_v_tilt_squ_1] -> cal sig/1(x)
  Constant100/1 -> Product1/1
  Abs1/1 -> Mux21/1
  Demux2/2 -> sigma_bar_v_tilt/2
  Integrator4/1 -> [d2_sigma_bar_v_hat], Out3/1
  [sigma_bar_v_tilt_squ_4] -> cal sig4/1(x)
  Abs5/1 -> Mux20/1
  Constant98/1 -> Mux19/3
  Constant111/1 -> Add1/1
  [sigma_bar_v_tilt] -> cal sig5/2(y)
  Constant109/1 -> Mux23/2
  [sigma_bar_v_tilt] -> Abs/1
  Mux24/1 -> Interpreted MATLAB Function23/1
  [sigma_bar_v_tilt] -> Abs1/1
  [sigma_bar_v_tilt_squ_5] -> cal sig5/1(x)
  Add1/1 -> Mux24/2
  cal sig4/1(z) -> [sigma_bar_v_sig_4]
  Constant161/1 -> Add/2
  [sigma_bar_v_tilt] -> cal sig3/2(y)
  Mux21/1 -> Interpreted MATLAB Function21/1
  Interpreted MATLAB Function22/1 -> trans to column23/1(x)
  Mux20/1 -> Interpreted MATLAB Function20/1
  x/1 -> choose sigma_bar_v/1(x)
  Constant105/1 -> Add/1
  Integrator2/1 -> [sigma_bar_v_hat], Out1/1
  Integrator3/1 -> [d_sigma_bar_v_hat], Out2/1

== matlab function sim_tcyb_2024_pos_ctrl/depart Re2 ==
  data: y output; x input
function y = fcn(x)
y = x(:,:,2);

end

== matlab function sim_tcyb_2024_pos_ctrl/depart Re3 ==
  data: y output; x input
function y = fcn(x)
y = x(:,:,3);

end

== matlab function sim_tcyb_2024_pos_ctrl/depart Re4 ==
  data: y output; x input
function y = fcn(x)
y = x(:,:,4);

end

== matlab function sim_tcyb_2024_pos_ctrl/cal differentiator d_sigma_bar_v_hat agent 3/cal sig1 ==
  data: x input; z output; y input
function z = fcn(x, y)
z = x(:) .* sign(y(:));

== matlab function sim_tcyb_2024_pos_ctrl/cal differentiator d_sigma_bar_v_hat agent 3/cal sig2 ==
  data: x input; z output; y input
function z = fcn(x, y)
z = x(:) .* sign(y(:));

== matlab function sim_tcyb_2024_pos_ctrl/cal differentiator d_sigma_bar_v_hat agent 3/cal sig3 ==
  data: x input; z output; y input
function z = fcn(x, y)
z = x(:) .* sign(y(:));

== matlab function sim_tcyb_2024_pos_ctrl/cal differentiator d_sigma_bar_v_hat agent 3/cal sig4 ==
  data: x input; z output; y input
function z = fcn(x, y)
z = x(:) .* sign(y(:));

== matlab function sim_tcyb_2024_pos_ctrl/generate translational disturbance agent 4 ==
  data: dp_aa_t input; dp_ff_t input; dp_phi_t input; dp_4 output; t input
function dp_4 = fcn(dp_aa_t, dp_ff_t, dp_phi_t, t)
%%%% 平移动力学方程中的扰动项设置
epsil_t = zeros(3, 1);

for kk = 1:5
    epsil_t = epsil_t + dp_aa_t(:, kk) .* sin( 2 * pi * dp_ff_t(:, kk) * t + dp_phi_t(:, kk) );
end

dp_4 = [ epsil_t(1) + 1.6 * sin( 0.2 * t ) + 2.0 * cos( 0.3 * t ) + 1.4 * sin( 0.5 * t ) ...
                + 4 * exp( -0.1 * t ) * sin( 0.5 * t ) + 3 / ( 1 + exp( -0.2 * ( t - 15 ) ) ); ...
                epsil_t(2) + 1.2 * sin( 0.1 * t ) + 3 * cos( 0.2 * t ) + 0.8 * sin( 0.4 * t ) ...
                + 2 * exp( -0.15 * t ) * cos( 0.6 * t ) + 3 / ( 1 + exp( -0.3 * ( t - 25 ) ) ); ...
                epsil_t(3) + 1.8 * sin( 0.1 * t ) + 1.6 * sin( 0.2 * t ) + 1.6 * cos( 0.3 * t ) ...
                + 4 * exp( -0.05 * t ) * sin( 0.4 * t + pi / 4 ) + 3 / ( 1 + exp( -0.5 * ( t - 20 ) ) ) ];

== matlab function sim_tcyb_2024_pos_ctrl/cal differentiator d_sigma_bar_v_hat agent 3/cal sig5 ==
  data: x input; z output; y input
function z = fcn(x, y)
z = x(:) .* sign(y(:));

== matlab function sim_tcyb_2024_pos_ctrl/cal differentiator d_sigma_bar_v_hat agent 3/choose sigma_bar_v ==
  data: x input; y output
function y = fcn(x)
iiuav = 3;
y = x(:,iiuav);

== matlab function sim_tcyb_2024_pos_ctrl/cal differentiator d_sigma_bar_v_hat agent 3/trans to column20 ==
  data: x input; y output
function y = fcn(x)
y = x(:);

== matlab function sim_tcyb_2024_pos_ctrl/cal differentiator d_sigma_bar_v_hat agent 3/trans to column21 ==
  data: x input; y output
function y = fcn(x)
y = x(:);

== matlab function sim_tcyb_2024_pos_ctrl/cal differentiator d_sigma_bar_v_hat agent 3/trans to column22 ==
  data: x input; y output
function y = fcn(x)
y = x(:);

== matlab function sim_tcyb_2024_pos_ctrl/cal differentiator d_sigma_bar_v_hat agent 3/trans to column23 ==
  data: x input; y output
function y = fcn(x)
y = x(:);

== matlab function sim_tcyb_2024_pos_ctrl/cal differentiator d_sigma_bar_v_hat agent 3/trans to column24 ==
  data: x input; y output
function y = fcn(x)
y = x(:);

== matlab function sim_tcyb_2024_pos_ctrl/cal differentiator d_sigma_bar_v_hat agent 3/trans to column25 ==
  data: x input; y output
function y = fcn(x)
y = x(:);

== matlab function sim_tcyb_2024_pos_ctrl/cal differentiator d_sigma_bar_v_hat agent 4/cal differentiator ==
  data: c1 input; d_sigma_bar_v_hat output; d_dsigma_bar_v_hat output; d_d2sigma_bar_v_hat output; c2 input; c3 input; chi_t input; sigma_bar_v_sig_1 input; sigma_bar_v_sig_2 input; sigma_bar_v_sig_3 input; sigma_bar_v_sig_4 input; sigma_bar_v_sig_5 input; sigma_bar_v_sig_6 input; d_sigma_bar_v_hat input; d2_sigma_bar_v_hat input
function [d_sigma_bar_v_hat, d_dsigma_bar_v_hat, d_d2sigma_bar_v_hat] = fcn(c1, c2, c3, chi_t, sigma_bar_v_sig_1, sigma_bar_v_sig_2, sigma_bar_v_sig_3, ...
                                                                                                                                                sigma_bar_v_sig_4, sigma_bar_v_sig_5, sigma_bar_v_sig_6, d_sigma_bar_v_hat, d2_sigma_bar_v_hat)
d_d2sigma_bar_v_hat = -chi_t .* c1 * sigma_bar_v_sig_1(:) - (1 - chi_t) .* c1 * sigma_bar_v_sig_2(:);
d_dsigma_bar_v_hat = -chi_t .* c2 * sigma_bar_v_sig_3(:) - (1 - chi_t) .* c2 * sigma_bar_v_sig_4(:) + d2_sigma_bar_v_hat(:);
d_sigma_bar_v_hat = -chi_t .* c3 * sigma_bar_v_sig_5(:) - (1 - chi_t) .* c3 * sigma_bar_v_sig_6(:) + d_sigma_bar_v_hat(:);

== matlab function sim_tcyb_2024_pos_ctrl/cal differentiator d_sigma_bar_v_hat agent 4/cal sig ==
  data: x input; z output; y input
function z = fcn(x, y)
z = x(:) .* sign(y(:));

== matlab function sim_tcyb_2024_pos_ctrl/cal differentiator d_sigma_bar_v_hat agent 4/cal sig1 ==
  data: x input; z output; y input
function z = fcn(x, y)
z = x(:) .* sign(y(:));

== matlab function sim_tcyb_2024_pos_ctrl/cal differentiator d_sigma_bar_v_hat agent 4/cal sig2 ==
  data: x input; z output; y input
function z = fcn(x, y)
z = x(:) .* sign(y(:));

== matlab function sim_tcyb_2024_pos_ctrl/desire formation position and velocity ==
  data: ksi0 input; eta0 input; delta_ksi_vec input; delta_eta_vec input; pos_i_des output; vel_i_des output
function [pos_i_des, vel_i_des] = fcn(ksi0, eta0, delta_ksi_vec, delta_eta_vec)
pos_i_des = zeros(3, 5);
vel_i_des = zeros(3, 5);
for iiuav = 1:5
    pos_i_des(:, iiuav) = ksi0(:) + delta_ksi_vec(:, iiuav);
    vel_i_des(:, iiuav) = eta0(:) + delta_eta_vec(:, iiuav);
end

== matlab function sim_tcyb_2024_pos_ctrl/cal differentiator d_sigma_bar_v_hat agent 4/cal sig3 ==
  data: x input; z output; y input
function z = fcn(x, y)
z = x(:) .* sign(y(:));

== matlab function sim_tcyb_2024_pos_ctrl/cal differentiator d_sigma_bar_v_hat agent 4/cal sig4 ==
  data: x input; z output; y input
function z = fcn(x, y)
z = x(:) .* sign(y(:));

== matlab function sim_tcyb_2024_pos_ctrl/cal differentiator d_sigma_bar_v_hat agent 4/cal sig5 ==
  data: x input; z output; y input
function z = fcn(x, y)
z = x(:) .* sign(y(:));

== matlab function sim_tcyb_2024_pos_ctrl/cal differentiator d_sigma_bar_v_hat agent 4/choose sigma_bar_v ==
  data: x input; y output
function y = fcn(x)
iiuav = 4;
y = x(:,iiuav);

== matlab function sim_tcyb_2024_pos_ctrl/cal differentiator d_sigma_bar_v_hat agent 4/trans to column20 ==
  data: x input; y output
function y = fcn(x)
y = x(:);

== matlab function sim_tcyb_2024_pos_ctrl/cal differentiator d_sigma_bar_v_hat agent 4/trans to column21 ==
  data: x input; y output
function y = fcn(x)
y = x(:);

== matlab function sim_tcyb_2024_pos_ctrl/cal differentiator d_sigma_bar_v_hat agent 4/trans to column22 ==
  data: x input; y output
function y = fcn(x)
y = x(:);

== matlab function sim_tcyb_2024_pos_ctrl/cal differentiator d_sigma_bar_v_hat agent 4/trans to column23 ==
  data: x input; y output
function y = fcn(x)
y = x(:);

== matlab function sim_tcyb_2024_pos_ctrl/cal Rci from ui ==
  data: Rci output; mi input; ui input
function Rci = fcn(mi, ui)
Rci = zeros(3,3,5);
for iiuav = 1:5
    Rci(:,:,iiuav) = cal_Rc_with_u(mi(iiuav), ui(:,iiuav));
end

end

== matlab function sim_tcyb_2024_pos_ctrl/cal differentiator d_sigma_bar_v_hat agent 4/trans to column24 ==
  data: x input; y output
function y = fcn(x)
y = x(:);

== matlab function sim_tcyb_2024_pos_ctrl/cal differentiator d_sigma_bar_v_hat agent 4/trans to column25 ==
  data: x input; y output
function y = fcn(x)
y = x(:);

== matlab function sim_tcyb_2024_pos_ctrl/cal differentiator d_sigma_bar_v_hat agent 5/cal differentiator ==
  data: c1 input; d_sigma_bar_v_hat output; d_dsigma_bar_v_hat output; d_d2sigma_bar_v_hat output; c2 input; c3 input; chi_t input; sigma_bar_v_sig_1 input; sigma_bar_v_sig_2 input; sigma_bar_v_sig_3 input; sigma_bar_v_sig_4 input; sigma_bar_v_sig_5 input; sigma_bar_v_sig_6 input; d_sigma_bar_v_hat input; d2_sigma_bar_v_hat input
function [d_sigma_bar_v_hat, d_dsigma_bar_v_hat, d_d2sigma_bar_v_hat] = fcn(c1, c2, c3, chi_t, sigma_bar_v_sig_1, sigma_bar_v_sig_2, sigma_bar_v_sig_3, ...
                                                                                                                                                sigma_bar_v_sig_4, sigma_bar_v_sig_5, sigma_bar_v_sig_6, d_sigma_bar_v_hat, d2_sigma_bar_v_hat)
d_d2sigma_bar_v_hat = -chi_t .* c1 * sigma_bar_v_sig_1(:) - (1 - chi_t) .* c1 * sigma_bar_v_sig_2(:);
d_dsigma_bar_v_hat = -chi_t .* c2 * sigma_bar_v_sig_3(:) - (1 - chi_t) .* c2 * sigma_bar_v_sig_4(:) + d2_sigma_bar_v_hat(:);
d_sigma_bar_v_hat = -chi_t .* c3 * sigma_bar_v_sig_5(:) - (1 - chi_t) .* c3 * sigma_bar_v_sig_6(:) + d_sigma_bar_v_hat(:);

== matlab function sim_tcyb_2024_pos_ctrl/cal differentiator d_sigma_bar_v_hat agent 5/cal sig ==
  data: x input; z output; y input
function z = fcn(x, y)
z = x(:) .* sign(y(:));

== matlab function sim_tcyb_2024_pos_ctrl/generate translational disturbance agent 5 ==
  data: dp_aa_t input; dp_ff_t input; dp_phi_t input; dp_5 output; t input
function dp_5 = fcn(dp_aa_t, dp_ff_t, dp_phi_t, t)
%%%% 平移动力学方程中的扰动项设置
epsil_t = zeros(3, 1);

for kk = 1:5
    epsil_t = epsil_t + dp_aa_t(:, kk) .* sin( 2 * pi * dp_ff_t(:, kk) * t + dp_phi_t(:, kk) );
end

dp_5 = [ epsil_t(1) + 1.6 * sin( 0.2 * t ) + 2.0 * cos( 0.3 * t ) + 1.4 * sin( 0.5 * t ) ...
                + 4 * exp( -0.1 * t ) * sin( 0.5 * t ) + 3 / ( 1 + exp( -0.2 * ( t - 15 ) ) ); ...
                epsil_t(2) + 1.2 * sin( 0.1 * t ) + 3 * cos( 0.2 * t ) + 0.8 * sin( 0.4 * t ) ...
                + 2 * exp( -0.15 * t ) * cos( 0.6 * t ) + 3 / ( 1 + exp( -0.3 * ( t - 25 ) ) ); ...
                epsil_t(3) + 1.8 * sin( 0.1 * t ) + 1.6 * sin( 0.2 * t ) + 1.6 * cos( 0.3 * t ) ...
                + 4 * exp( -0.05 * t ) * sin( 0.4 * t + pi / 4 ) + 3 / ( 1 + exp( -0.5 * ( t - 20 ) ) ) ];

== matlab function sim_tcyb_2024_pos_ctrl/cal differentiator d_sigma_bar_v_hat agent 5/cal sig1 ==
  data: x input; z output; y input
function z = fcn(x, y)
z = x(:) .* sign(y(:));

== matlab function sim_tcyb_2024_pos_ctrl/cal differentiator d_sigma_bar_v_hat agent 5/cal sig2 ==
  data: x input; z output; y input
function z = fcn(x, y)
z = x(:) .* sign(y(:));

== matlab function sim_tcyb_2024_pos_ctrl/cal differentiator d_sigma_bar_v_hat agent 5/cal sig3 ==
  data: x input; z output; y input
function z = fcn(x, y)
z = x(:) .* sign(y(:));

== matlab function sim_tcyb_2024_pos_ctrl/cal differentiator d_sigma_bar_v_hat agent 5/cal sig4 ==
  data: x input; z output; y input
function z = fcn(x, y)
z = x(:) .* sign(y(:));

== matlab function sim_tcyb_2024_pos_ctrl/cal differentiator d_sigma_bar_v_hat agent 5/cal sig5 ==
  data: x input; z output; y input
function z = fcn(x, y)
z = x(:) .* sign(y(:));

== matlab function sim_tcyb_2024_pos_ctrl/cal differentiator d_sigma_bar_v_hat agent 5/choose sigma_bar_v ==
  data: x input; y output
function y = fcn(x)
iiuav = 5;
y = x(:,iiuav);

== matlab function sim_tcyb_2024_pos_ctrl/cal differentiator d_sigma_bar_v_hat agent 5/trans to column20 ==
  data: x input; y output
function y = fcn(x)
y = x(:);

== matlab function sim_tcyb_2024_pos_ctrl/cal differentiator d_sigma_bar_v_hat agent 5/trans to column21 ==
  data: x input; y output
function y = fcn(x)
y = x(:);

== matlab function sim_tcyb_2024_pos_ctrl/cal differentiator d_sigma_bar_v_hat agent 5/trans to column22 ==
  data: x input; y output
function y = fcn(x)
y = x(:);

== matlab function sim_tcyb_2024_pos_ctrl/cal differentiator d_sigma_bar_v_hat agent 5/trans to column23 ==
  data: x input; y output
function y = fcn(x)
y = x(:);

== matlab function sim_tcyb_2024_pos_ctrl/cal differentiator d_sigma_bar_v_hat agent 5/trans to column24 ==
  data: x input; y output
function y = fcn(x)
y = x(:);

== matlab function sim_tcyb_2024_pos_ctrl/cal differentiator d_sigma_bar_v_hat agent 5/trans to column25 ==
  data: x input; y output
function y = fcn(x)
y = x(:);

== matlab function sim_tcyb_2024_pos_ctrl/combine d_sigma_bar_v_est ==
  data: d_sigma_bar_v_est_1 input; d_sigma_bar_v_est_2 input; d_sigma_bar_v_est_3 input; d_sigma_bar_v_est_4 input; d_sigma_bar_v_est_5 input; d_sigma_bar_v_vec output
function d_sigma_bar_v_vec  = fcn(d_sigma_bar_v_est_1, d_sigma_bar_v_est_2, d_sigma_bar_v_est_3, d_sigma_bar_v_est_4, d_sigma_bar_v_est_5)
%%%% 合并用微分器求得的虚拟速度控制量导数
d_sigma_bar_v_vec = [d_sigma_bar_v_est_1(:), d_sigma_bar_v_est_2(:), d_sigma_bar_v_est_3(:), d_sigma_bar_v_est_4(:), d_sigma_bar_v_est_5(:)];

== matlab function sim_tcyb_2024_pos_ctrl/combine translational disturbance ==
  data: dp_vec output; dp_1 input; dp_2 input; dp_3 input; dp_4 input; dp_5 input
function dp_vec = fcn(dp_1, dp_2, dp_3, dp_4, dp_5)
%%%% 合并领导者编队跟踪误差结果
dp_vec = [dp_1(:), dp_2(:), dp_3(:), dp_4(:), dp_5(:)];

== matlab function sim_tcyb_2024_pos_ctrl/cal abs 21 ==
  data: x input; y output
function y = fcn(x)
y = abs(x(:));

== matlab function sim_tcyb_2024_pos_ctrl/cal abs 22 ==
  data: x input; y output
function y = fcn(x)
y = abs(x(:));

== matlab function sim_tcyb_2024_pos_ctrl/choose ksi_est_err 21 ==
  data: x input; y output
function y = fcn(x)
iiuav = 1;
y = x(:,iiuav);

== matlab function sim_tcyb_2024_pos_ctrl/choose ksi_est_err 22 ==
  data: x input; y output
function y = fcn(x)
iiuav = 1;
y = x(:,iiuav);

== matlab function sim_tcyb_2024_pos_ctrl/trans to column20 ==
  data: x input; y output
function y = fcn(x)
y = x(:);

== matlab function sim_tcyb_2024_pos_ctrl/trans to column21 ==
  data: x input; y output
function y = fcn(x)
y = x(:);

== matlab function sim_tcyb_2024_pos_ctrl/cal theta_sigma_bar_v_tilt agent 1 ==
  data: alfa_theta input; sigma_bar_v_tilt_squ_1_1 input; theta_sigma_bar_v_tilt_1_1 output; sigma_bar_v_tilt_squ_2_1 input; sigma_bar_v_tilt_vec input; theta_sigma_bar_v_tilt_2_1 output
function [theta_sigma_bar_v_tilt_1_1, theta_sigma_bar_v_tilt_2_1] = fcn(alfa_theta, sigma_bar_v_tilt_squ_1_1, sigma_bar_v_tilt_squ_2_1, sigma_bar_v_tilt_vec)
%%%% 计算平滑递增函数
iiuav = 1;
theta_sigma_bar_v_tilt_1_1 = sigma_bar_v_tilt_squ_1_1(:) .* ( -1 + 2 ./ ( 1 + exp( -alfa_theta .* sigma_bar_v_tilt_vec(:,iiuav) ) ) );
theta_sigma_bar_v_tilt_2_1 = sigma_bar_v_tilt_squ_2_1(:) .* ( -1 + 2 ./ ( 1 + exp( -alfa_theta .* sigma_bar_v_tilt_vec(:,iiuav) ) ) );

== matlab function sim_tcyb_2024_pos_ctrl/cal abs 23 ==
  data: x input; y output
function y = fcn(x)
y = abs(x(:));

== matlab function sim_tcyb_2024_pos_ctrl/cal abs 24 ==
  data: x input; y output
function y = fcn(x)
y = abs(x(:));

== matlab function sim_tcyb_2024_pos_ctrl/cal theta_sigma_bar_v_tilt agent 2 ==
  data: alfa_theta input; sigma_bar_v_tilt_squ_1_2 input; theta_sigma_bar_v_tilt_1_2 output; sigma_bar_v_tilt_squ_2_2 input; sigma_bar_v_tilt_vec input; theta_sigma_bar_v_tilt_2_2 output
function [theta_sigma_bar_v_tilt_1_2, theta_sigma_bar_v_tilt_2_2] = fcn(alfa_theta, sigma_bar_v_tilt_squ_1_2, sigma_bar_v_tilt_squ_2_2, sigma_bar_v_tilt_vec)
%%%% 计算平滑递增函数
iiuav = 2;
theta_sigma_bar_v_tilt_1_2 = sigma_bar_v_tilt_squ_1_2(:) .* ( -1 + 2 ./ ( 1 + exp( -alfa_theta .* sigma_bar_v_tilt_vec(:,iiuav) ) ) );
theta_sigma_bar_v_tilt_2_2 = sigma_bar_v_tilt_squ_2_2(:) .* ( -1 + 2 ./ ( 1 + exp( -alfa_theta .* sigma_bar_v_tilt_vec(:,iiuav) ) ) );

== matlab function sim_tcyb_2024_pos_ctrl/choose ksi_est_err 23 ==
  data: x input; y output
function y = fcn(x)
iiuav = 2;
y = x(:,iiuav);

== matlab function sim_tcyb_2024_pos_ctrl/choose ksi_est_err 24 ==
  data: x input; y output
function y = fcn(x)
iiuav = 2;
y = x(:,iiuav);

== matlab function sim_tcyb_2024_pos_ctrl/trans to column22 ==
  data: x input; y output
function y = fcn(x)
y = x(:);

== matlab function sim_tcyb_2024_pos_ctrl/trans to column23 ==
  data: x input; y output
function y = fcn(x)
y = x(:);

== matlab function sim_tcyb_2024_pos_ctrl/cal formation tracking velocity errors ==
  data: wi0 input; err_eta_form_vec output; wij input; err_eta_vec input
function err_eta_form_vec = fcn(wi0, wij, err_eta_vec)
%%%% 计算编队跟踪误差
err_eta_form_vec = zeros(3,5);
for iiuav = 1:5
    err_eta_form_vec(:,iiuav) = wi0(iiuav, iiuav) * err_eta_vec(:,iiuav);
    for jjuav = 1:5
        err_eta_form_vec(:,iiuav) = err_eta_form_vec(:,iiuav) ...
                                                        + wij(iiuav, jjuav) * (err_eta_vec(:,iiuav) - err_eta_vec(:,jjuav));
    end
end

== matlab function sim_tcyb_2024_pos_ctrl/cal abs 25 ==
  data: x input; y output
function y = fcn(x)
y = abs(x(:));

== matlab function sim_tcyb_2024_pos_ctrl/cal abs 26 ==
  data: x input; y output
function y = fcn(x)
y = abs(x(:));
